simulink model "Quadcopter_nonlinear"  (R2023a)
settings: Solver=ode4  StartTime=0.0  StopTime=0.2  FixedStep=0.02  RelTol=1e-3
values from neighbouring files (symbols this model uses):
  b = 1.10794e-5    (= 1.10794e-05)    [QuadParameter.m]
  d = 3.2e-6    (= 3.2e-06)    [QuadParameter.m]
  d_cg = 0.295    [QuadParameter.m]
  Gamma1 = 4.98954110218396e-06    (= 4.98954110218e-06)    [final_PS.m]
  Gamma10 = -1.44562619785504e-05    (= -1.44562619786e-05)    [final_PS.m]
  Gamma11 = 24.4566929368231    (= 24.4566929368)    [final_PS.m]
  Gamma2 = 0.00290613207976024    (= 0.00290613207976)    [final_PS.m]
  Gamma3 = 42.1805100768496    (= 42.1805100768)    [final_PS.m]
  Gamma4 = 0.000237183411278011    (= 0.000237183411278)    [final_PS.m]
  Gamma5 = -0.00234577516229748    (= -0.0023457751623)    [final_PS.m]
  Gamma6 = 2.52935414320957    (= 2.52935414321)    [final_PS.m]
  Gamma7 = 0.000224057181768728    (= 0.000224057181769)    [final_PS.m]
  Gamma8 = 18.4688604256806    (= 18.4688604257)    [final_PS.m]
  Gamma9 = 0.00216966508125569    (= 0.00216966508126)    [final_PS.m]
  init_I = data_I(1, :)    [PS_I.m]
  init_II = data_II(1, :)    [PS_II.m]
  init_III = data_III(1, :)    [PS_III.m]
  init_IV = data_IV(1, :)    [PS_IV.m]
  init_IX = data_IX(1, :)    [PS_IX.m]
  init_V = data_V(1, :)    [PS_V.m]
  init_VI = data_VI(1, :)    [PS_VI.m]
  Omega_I = Omega(1, :)    [PS_I.m]
  Omega_II = Omega(1, :)    [PS_II.m]
  Omega_III = Omega(1, :)    [PS_III.m]
  Omega_IV = Omega(1, :)    [PS_IV.m]
  Omega_IX = Omega(1, :)    [PS_IX.m]
  Omega_V = Omega(1, :)    [PS_V.m]
  Omega_VI = Omega(1, :)    [PS_VI.m]
  Omega_VII = Omega(1, :)    [PS_VII.m]
  Omega_VIII = Omega(1, :)    [PS_VIII.m]
  Omega_X = Omega(1, :)    [PS_X.m]
undefined symbols (not defined in the file or in its folder): init_VII, init_VIII, init_X
(part 1 of 3)
settings Model: Creator=Ali  LastModifiedBy=Ali
settings SolverCC: AlgebraicLoopSolver=TrustRegion
settings OptimizationCC: ReuseModelBlockBuffer=off
settings DebuggingCC: UnconnectedInputMsg=warning  UnconnectedOutputMsg=warning  UnconnectedLineMsg=warning
settings ModelReferenceCC: EnableRefExpFcnMdlSchedulingChecks=on

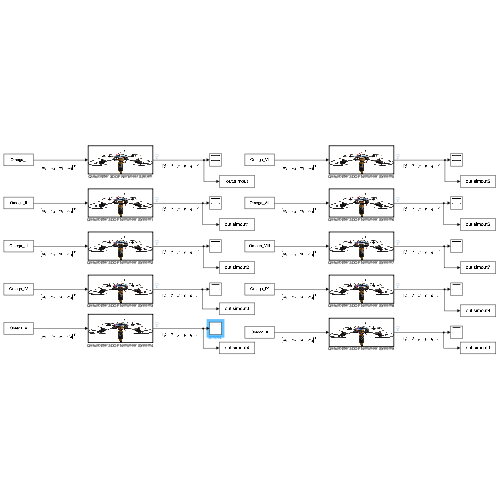
[thumbnail: Simulink's stored preview of the top-level diagram]
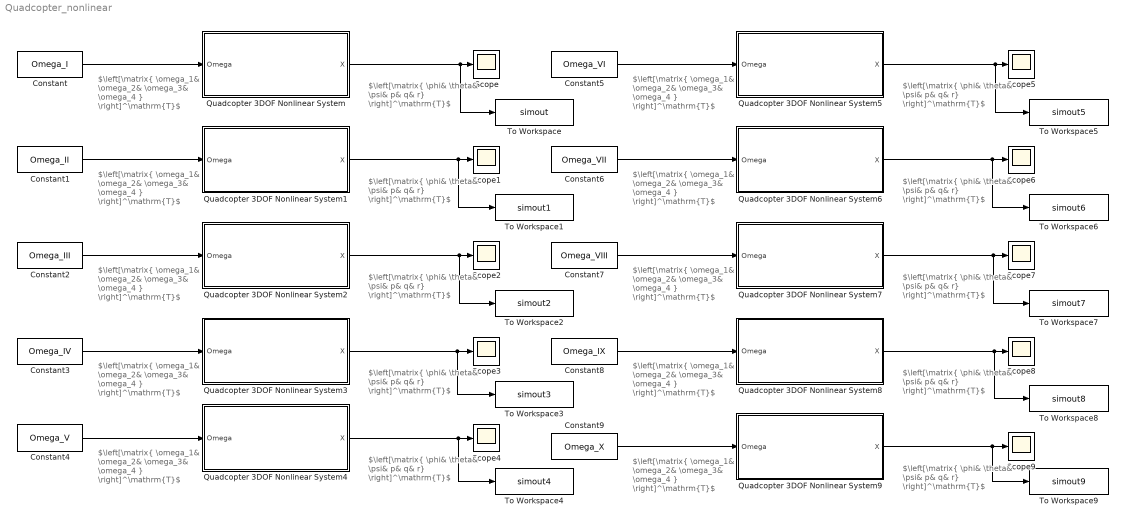
== system Quadcopter_nonlinear ==
  note: $\left[\matrix{ \omega_1& \omega_2& \omega_3& \omega_4 } \right]^\mathrm{T}$
  note: $\left[\matrix{ \phi& \theta& \psi& p& q& r} \right]^\mathrm{T}$
  note: $\left[\matrix{ \phi& \theta& \psi& p& q& r} \right]^\mathrm{T}$
  note: $\left[\matrix{ \omega_1& \omega_2& \omega_3& \omega_4 } \right]^\mathrm{T}$
  note: $\left[\matrix{ \phi& \theta& \psi& p& q& r} \right]^\mathrm{T}$
  note: $\left[\matrix{ \omega_1& \omega_2& \omega_3& \omega_4 } \right]^\mathrm{T}$
  note: $\left[\matrix{ \omega_1& \omega_2& \omega_3& \omega_4 } \right]^\mathrm{T}$
  note: $\left[\matrix{ \phi& \theta& \psi& p& q& r} \right]^\mathrm{T}$
  note: $\left[\matrix{ \phi& \theta& \psi& p& q& r} \right]^\mathrm{T}$
  note: $\left[\matrix{ \omega_1& \omega_2& \omega_3& \omega_4 } \right]^\mathrm{T}$
  note: $\left[\matrix{ \phi& \theta& \psi& p& q& r} \right]^\mathrm{T}$
  note: $\left[\matrix{ \phi& \theta& \psi& p& q& r} \right]^\mathrm{T}$
  note: $\left[\matrix{ \omega_1& \omega_2& \omega_3& \omega_4 } \right]^\mathrm{T}$
  note: $\left[\matrix{ \phi& \theta& \psi& p& q& r} \right]^\mathrm{T}$
  note: $\left[\matrix{ \phi& \theta& \psi& p& q& r} \right]^\mathrm{T}$
  note: $\left[\matrix{ \omega_1& \omega_2& \omega_3& \omega_4 } \right]^\mathrm{T}$
  note: $\left[\matrix{ \omega_1& \omega_2& \omega_3& \omega_4 } \right]^\mathrm{T}$
  note: $\left[\matrix{ \omega_1& \omega_2& \omega_3& \omega_4 } \right]^\mathrm{T}$
  note: $\left[\matrix{ \phi& \theta& \psi& p& q& r} \right]^\mathrm{T}$
  note: $\left[\matrix{ \omega_1& \omega_2& \omega_3& \omega_4 } \right]^\mathrm{T}$
  Constant : Constant  Value=Omega_I
  Constant1 : Constant  Value=Omega_II
  Constant2 : Constant  Value=Omega_III
  Constant3 : Constant  Value=Omega_IV
  Constant4 : Constant  Value=Omega_V
  Constant5 : Constant  Value=Omega_VI
  Constant6 : Constant  Value=Omega_VII
  Constant7 : Constant  Value=Omega_VIII
  Constant8 : Constant  Value=Omega_IX
  Constant9 : Constant  Value=Omega_X
  Quadcopter 3DOF Nonlinear System : Subsystem  TreatAsAtomicUnit=on
      mask Display: image('quad1.png'); % Use "Edit Image" on toolstrip to change.
  Quadcopter 3DOF Nonlinear System1 : Subsystem  TreatAsAtomicUnit=on
      mask Display: image('quad1.png'); % Use "Edit Image" on toolstrip to change.
  Quadcopter 3DOF Nonlinear System2 : Subsystem  TreatAsAtomicUnit=on
      mask Display: image('quad1.png'); % Use "Edit Image" on toolstrip to change.
  Quadcopter 3DOF Nonlinear System3 : Subsystem  TreatAsAtomicUnit=on
      mask Display: image('quad1.png'); % Use "Edit Image" on toolstrip to change.
  Quadcopter 3DOF Nonlinear System4 : Subsystem  TreatAsAtomicUnit=on
      mask Display: image('quad1.png'); % Use "Edit Image" on toolstrip to change.
  Quadcopter 3DOF Nonlinear System5 : Subsystem  TreatAsAtomicUnit=on
      mask Display: image('quad1.png'); % Use "Edit Image" on toolstrip to change.
  Quadcopter 3DOF Nonlinear System6 : Subsystem  TreatAsAtomicUnit=on
      mask Display: image('quad1.png'); % Use "Edit Image" on toolstrip to change.
  Quadcopter 3DOF Nonlinear System7 : Subsystem  TreatAsAtomicUnit=on
      mask Display: image('quad1.png'); % Use "Edit Image" on toolstrip to change.
  Quadcopter 3DOF Nonlinear System8 : Subsystem  TreatAsAtomicUnit=on
      mask Display: image('quad1.png'); % Use "Edit Image" on toolstrip to change.
  Quadcopter 3DOF Nonlinear System9 : Subsystem  TreatAsAtomicUnit=on
      mask Display: image('quad1.png'); % Use "Edit Image" on toolstrip to change.
  Scope{,1..9} (10 alike) : Scope
  To Workspace : ToWorkspace  VariableName=simout  SampleTime=-1
      settings: Save2DSignal=2-D array (concatenate along first dimension)
  To Workspace1 : ToWorkspace  VariableName=simout1  SampleTime=-1
      settings: Save2DSignal=2-D array (concatenate along first dimension)
  To Workspace2 : ToWorkspace  VariableName=simout2  SampleTime=-1
      settings: Save2DSignal=2-D array (concatenate along first dimension)
  To Workspace3 : ToWorkspace  VariableName=simout3  SampleTime=-1
      settings: Save2DSignal=2-D array (concatenate along first dimension)
  To Workspace4 : ToWorkspace  VariableName=simout4  SampleTime=-1
      settings: Save2DSignal=2-D array (concatenate along first dimension)
  To Workspace5 : ToWorkspace  VariableName=simout5  SampleTime=-1
      settings: Save2DSignal=2-D array (concatenate along first dimension)
  To Workspace6 : ToWorkspace  VariableName=simout6  SampleTime=-1
      settings: Save2DSignal=2-D array (concatenate along first dimension)
  To Workspace7 : ToWorkspace  VariableName=simout7  SampleTime=-1
      settings: Save2DSignal=2-D array (concatenate along first dimension)
  To Workspace8 : ToWorkspace  VariableName=simout8  SampleTime=-1
      settings: Save2DSignal=2-D array (concatenate along first dimension)
  To Workspace9 : ToWorkspace  VariableName=simout9  SampleTime=-1
      settings: Save2DSignal=2-D array (concatenate along first dimension)
  wires:
  Constant/1 -> Quadcopter 3DOF Nonlinear System/1(Omega)
  Quadcopter 3DOF Nonlinear System/1(X) -> To Workspace/1, Scope/1
  Constant1/1 -> Quadcopter 3DOF Nonlinear System1/1(Omega)
  Quadcopter 3DOF Nonlinear System1/1(X) -> To Workspace1/1, Scope1/1
  Constant2/1 -> Quadcopter 3DOF Nonlinear System2/1(Omega)
  Quadcopter 3DOF Nonlinear System2/1(X) -> To Workspace2/1, Scope2/1
  Quadcopter 3DOF Nonlinear System3/1(X) -> To Workspace3/1, Scope3/1
  Constant3/1 -> Quadcopter 3DOF Nonlinear System3/1(Omega)
  Quadcopter 3DOF Nonlinear System4/1(X) -> To Workspace4/1, Scope4/1
  Constant4/1 -> Quadcopter 3DOF Nonlinear System4/1(Omega)
  Constant5/1 -> Quadcopter 3DOF Nonlinear System5/1(Omega)
  Quadcopter 3DOF Nonlinear System8/1(X) -> To Workspace8/1, Scope8/1
  Quadcopter 3DOF Nonlinear System6/1(X) -> To Workspace6/1, Scope6/1
  Constant6/1 -> Quadcopter 3DOF Nonlinear System6/1(Omega)
  Quadcopter 3DOF Nonlinear System7/1(X) -> To Workspace7/1, Scope7/1
  Quadcopter 3DOF Nonlinear System5/1(X) -> To Workspace5/1, Scope5/1
  Constant7/1 -> Quadcopter 3DOF Nonlinear System7/1(Omega)
  Constant8/1 -> Quadcopter 3DOF Nonlinear System8/1(Omega)
  Quadcopter 3DOF Nonlinear System9/1(X) -> To Workspace9/1, Scope9/1
  Constant9/1 -> Quadcopter 3DOF Nonlinear System9/1(Omega)

== system Quadcopter_nonlinear/Quadcopter 3DOF Nonlinear System ==
  note: $\dot X$
  note: $\left[\matrix{ \dot\phi& \dot\theta& \dot\psi& \dot p& \dot q& \dot r} \right]^\mathrm{T}$
  note: $\left[\matrix{ \phi& \theta& \psi& p& q& r} \right]^\mathrm{T}$
  Omega : Inport
  Integrator : Integrator  InitialCondition=init_I
  Quad System1 : Subsystem
  X : Outport
  wires:
  Integrator/1 -> Quad System1/1(X), X/1  "X"
  Quad System1/1(dot(X)) -> Integrator/1  "dot(X)"
  Omega/1 -> Quad System1/2(Omega)

== system Quadcopter_nonlinear/Quadcopter 3DOF Nonlinear System1 ==
  note: $\dot X$
  note: $\left[\matrix{ \dot\phi& \dot\theta& \dot\psi& \dot p& \dot q& \dot r} \right]^\mathrm{T}$
  note: $\left[\matrix{ \phi& \theta& \psi& p& q& r} \right]^\mathrm{T}$
  Omega : Inport
  Integrator : Integrator  InitialCondition=init_II
  Quad System1 : Subsystem
  X : Outport
  wires:
  Integrator/1 -> Quad System1/1(X), X/1  "X"
  Quad System1/1(dot(X)) -> Integrator/1  "dot(X)"
  Omega/1 -> Quad System1/2(Omega)

== system Quadcopter_nonlinear/Quadcopter 3DOF Nonlinear System2 ==
  note: $\dot X$
  note: $\left[\matrix{ \dot\phi& \dot\theta& \dot\psi& \dot p& \dot q& \dot r} \right]^\mathrm{T}$
  note: $\left[\matrix{ \phi& \theta& \psi& p& q& r} \right]^\mathrm{T}$
  Omega : Inport
  Integrator : Integrator  InitialCondition=init_III
  Quad System1 : Subsystem
  X : Outport
  wires:
  Integrator/1 -> Quad System1/1(X), X/1  "X"
  Quad System1/1(dot(X)) -> Integrator/1  "dot(X)"
  Omega/1 -> Quad System1/2(Omega)

== system Quadcopter_nonlinear/Quadcopter 3DOF Nonlinear System3 ==
  note: $\dot X$
  note: $\left[\matrix{ \dot\phi& \dot\theta& \dot\psi& \dot p& \dot q& \dot r} \right]^\mathrm{T}$
  note: $\left[\matrix{ \phi& \theta& \psi& p& q& r} \right]^\mathrm{T}$
  Omega : Inport
  Integrator : Integrator  InitialCondition=init_IV
  Quad System1 : Subsystem
  X : Outport
  wires:
  Integrator/1 -> Quad System1/1(X), X/1  "X"
  Quad System1/1(dot(X)) -> Integrator/1  "dot(X)"
  Omega/1 -> Quad System1/2(Omega)

== system Quadcopter_nonlinear/Quadcopter 3DOF Nonlinear System4 ==
  note: $\dot X$
  note: $\left[\matrix{ \dot\phi& \dot\theta& \dot\psi& \dot p& \dot q& \dot r} \right]^\mathrm{T}$
  note: $\left[\matrix{ \phi& \theta& \psi& p& q& r} \right]^\mathrm{T}$
  Omega : Inport
  Integrator : Integrator  InitialCondition=init_V
  Quad System1 : Subsystem
  X : Outport
  wires:
  Integrator/1 -> Quad System1/1(X), X/1  "X"
  Quad System1/1(dot(X)) -> Integrator/1  "dot(X)"
  Omega/1 -> Quad System1/2(Omega)

== system Quadcopter_nonlinear/Quadcopter 3DOF Nonlinear System5 ==
  note: $\dot X$
  note: $\left[\matrix{ \dot\phi& \dot\theta& \dot\psi& \dot p& \dot q& \dot r} \right]^\mathrm{T}$
  note: $\left[\matrix{ \phi& \theta& \psi& p& q& r} \right]^\mathrm{T}$
  Omega : Inport
  Integrator : Integrator  InitialCondition=init_VI
  Quad System1 : Subsystem
  X : Outport
  wires:
  Integrator/1 -> Quad System1/1(X), X/1  "X"
  Quad System1/1(dot(X)) -> Integrator/1  "dot(X)"
  Omega/1 -> Quad System1/2(Omega)

== system Quadcopter_nonlinear/Quadcopter 3DOF Nonlinear System6 ==
  note: $\dot X$
  note: $\left[\matrix{ \dot\phi& \dot\theta& \dot\psi& \dot p& \dot q& \dot r} \right]^\mathrm{T}$
  note: $\left[\matrix{ \phi& \theta& \psi& p& q& r} \right]^\mathrm{T}$
  Omega : Inport
  Integrator : Integrator  InitialCondition=init_VII
  Quad System1 : Subsystem
  X : Outport
  wires:
  Integrator/1 -> Quad System1/1(X), X/1  "X"
  Quad System1/1(dot(X)) -> Integrator/1  "dot(X)"
  Omega/1 -> Quad System1/2(Omega)

== system Quadcopter_nonlinear/Quadcopter 3DOF Nonlinear System7 ==
  note: $\dot X$
  note: $\left[\matrix{ \dot\phi& \dot\theta& \dot\psi& \dot p& \dot q& \dot r} \right]^\mathrm{T}$
  note: $\left[\matrix{ \phi& \theta& \psi& p& q& r} \right]^\mathrm{T}$
  Omega : Inport
  Integrator : Integrator  InitialCondition=init_VIII
  Quad System1 : Subsystem
  X : Outport
  wires:
  Integrator/1 -> Quad System1/1(X), X/1  "X"
  Quad System1/1(dot(X)) -> Integrator/1  "dot(X)"
  Omega/1 -> Quad System1/2(Omega)

== system Quadcopter_nonlinear/Quadcopter 3DOF Nonlinear System8 ==
  note: $\dot X$
  note: $\left[\matrix{ \dot\phi& \dot\theta& \dot\psi& \dot p& \dot q& \dot r} \right]^\mathrm{T}$
  note: $\left[\matrix{ \phi& \theta& \psi& p& q& r} \right]^\mathrm{T}$
  Omega : Inport
  Integrator : Integrator  InitialCondition=init_IX
  Quad System1 : Subsystem
  X : Outport
  wires:
  Integrator/1 -> Quad System1/1(X), X/1  "X"
  Quad System1/1(dot(X)) -> Integrator/1  "dot(X)"
  Omega/1 -> Quad System1/2(Omega)

== system Quadcopter_nonlinear/Quadcopter 3DOF Nonlinear System9 ==
  note: $\dot X$
  note: $\left[\matrix{ \dot\phi& \dot\theta& \dot\psi& \dot p& \dot q& \dot r} \right]^\mathrm{T}$
  note: $\left[\matrix{ \phi& \theta& \psi& p& q& r} \right]^\mathrm{T}$
  Omega : Inport
  Integrator : Integrator  InitialCondition=init_X
  Quad System1 : Subsystem
  X : Outport
  wires:
  Integrator/1 -> Quad System1/1(X), X/1  "X"
  Quad System1/1(dot(X)) -> Integrator/1  "dot(X)"
  Omega/1 -> Quad System1/2(Omega)

== system Quadcopter_nonlinear/Quadcopter 3DOF Nonlinear System/Quad System1 ==
  X : Inport
  Omega : Inport  Port=2
  Quad System : Subsystem
  Selector : Selector  InputPortWidth=6  IndexOptions=Index vector (dialog)  Indices=[1 2 3 4 5 6]  OutputSizes=1
  Subsystem : Subsystem
  dot(X) : Outport
  wires:
  Selector/1 -> dot(X)/1  "dot(X)"
  X/1 -> Subsystem/1(X)
  Omega/1 -> Quad System/2(Omega)
  Quad System/1(dot(X)) -> Selector/1  "dot(X)"
  Subsystem/1(X_6) -> Quad System/1(X)

== system Quadcopter_nonlinear/Quadcopter 3DOF Nonlinear System1/Quad System1 ==
  X : Inport
  Omega : Inport  Port=2
  Quad System : Subsystem
  Selector : Selector  InputPortWidth=6  IndexOptions=Index vector (dialog)  Indices=[1 2 3 4 5 6]  OutputSizes=1
  Subsystem : Subsystem
  dot(X) : Outport
  wires:
  Selector/1 -> dot(X)/1  "dot(X)"
  X/1 -> Subsystem/1(X)
  Omega/1 -> Quad System/2(Omega)
  Quad System/1(dot(X)) -> Selector/1  "dot(X)"
  Subsystem/1(X_6) -> Quad System/1(X)

== system Quadcopter_nonlinear/Quadcopter 3DOF Nonlinear System2/Quad System1 ==
  X : Inport
  Omega : Inport  Port=2
  Quad System : Subsystem
  Selector : Selector  InputPortWidth=6  IndexOptions=Index vector (dialog)  Indices=[1 2 3 4 5 6]  OutputSizes=1
  Subsystem : Subsystem
  dot(X) : Outport
  wires:
  Selector/1 -> dot(X)/1  "dot(X)"
  X/1 -> Subsystem/1(X)
  Omega/1 -> Quad System/2(Omega)
  Quad System/1(dot(X)) -> Selector/1  "dot(X)"
  Subsystem/1(X_6) -> Quad System/1(X)

== system Quadcopter_nonlinear/Quadcopter 3DOF Nonlinear System3/Quad System1 ==
  X : Inport
  Omega : Inport  Port=2
  Quad System : Subsystem
  Selector : Selector  InputPortWidth=6  IndexOptions=Index vector (dialog)  Indices=[1 2 3 4 5 6]  OutputSizes=1
  Subsystem : Subsystem
  dot(X) : Outport
  wires:
  Selector/1 -> dot(X)/1  "dot(X)"
  X/1 -> Subsystem/1(X)
  Omega/1 -> Quad System/2(Omega)
  Quad System/1(dot(X)) -> Selector/1  "dot(X)"
  Subsystem/1(X_6) -> Quad System/1(X)

== system Quadcopter_nonlinear/Quadcopter 3DOF Nonlinear System4/Quad System1 ==
  X : Inport
  Omega : Inport  Port=2
  Quad System : Subsystem
  Selector : Selector  InputPortWidth=6  IndexOptions=Index vector (dialog)  Indices=[1 2 3 4 5 6]  OutputSizes=1
  Subsystem : Subsystem
  dot(X) : Outport
  wires:
  Selector/1 -> dot(X)/1  "dot(X)"
  X/1 -> Subsystem/1(X)
  Omega/1 -> Quad System/2(Omega)
  Quad System/1(dot(X)) -> Selector/1  "dot(X)"
  Subsystem/1(X_6) -> Quad System/1(X)

== system Quadcopter_nonlinear/Quadcopter 3DOF Nonlinear System5/Quad System1 ==
  X : Inport
  Omega : Inport  Port=2
  Quad System : Subsystem
  Selector : Selector  InputPortWidth=6  IndexOptions=Index vector (dialog)  Indices=[1 2 3 4 5 6]  OutputSizes=1
  Subsystem : Subsystem
  dot(X) : Outport
  wires:
  Selector/1 -> dot(X)/1  "dot(X)"
  X/1 -> Subsystem/1(X)
  Omega/1 -> Quad System/2(Omega)
  Quad System/1(dot(X)) -> Selector/1  "dot(X)"
  Subsystem/1(X_6) -> Quad System/1(X)

== system Quadcopter_nonlinear/Quadcopter 3DOF Nonlinear System6/Quad System1 ==
  X : Inport
  Omega : Inport  Port=2
  Quad System : Subsystem
  Selector : Selector  InputPortWidth=6  IndexOptions=Index vector (dialog)  Indices=[1 2 3 4 5 6]  OutputSizes=1
  Subsystem : Subsystem
  dot(X) : Outport
  wires:
  Selector/1 -> dot(X)/1  "dot(X)"
  X/1 -> Subsystem/1(X)
  Omega/1 -> Quad System/2(Omega)
  Quad System/1(dot(X)) -> Selector/1  "dot(X)"
  Subsystem/1(X_6) -> Quad System/1(X)

== system Quadcopter_nonlinear/Quadcopter 3DOF Nonlinear System7/Quad System1 ==
  X : Inport
  Omega : Inport  Port=2
  Quad System : Subsystem
  Selector : Selector  InputPortWidth=6  IndexOptions=Index vector (dialog)  Indices=[1 2 3 4 5 6]  OutputSizes=1
  Subsystem : Subsystem
  dot(X) : Outport
  wires:
  Selector/1 -> dot(X)/1  "dot(X)"
  X/1 -> Subsystem/1(X)
  Omega/1 -> Quad System/2(Omega)
  Quad System/1(dot(X)) -> Selector/1  "dot(X)"
  Subsystem/1(X_6) -> Quad System/1(X)

== system Quadcopter_nonlinear/Quadcopter 3DOF Nonlinear System8/Quad System1 ==
  X : Inport
  Omega : Inport  Port=2
  Quad System : Subsystem
  Selector : Selector  InputPortWidth=6  IndexOptions=Index vector (dialog)  Indices=[1 2 3 4 5 6]  OutputSizes=1
  Subsystem : Subsystem
  dot(X) : Outport
  wires:
  Selector/1 -> dot(X)/1  "dot(X)"
  X/1 -> Subsystem/1(X)
  Omega/1 -> Quad System/2(Omega)
  Quad System/1(dot(X)) -> Selector/1  "dot(X)"
  Subsystem/1(X_6) -> Quad System/1(X)

== system Quadcopter_nonlinear/Quadcopter 3DOF Nonlinear System9/Quad System1 ==
  X : Inport
  Omega : Inport  Port=2
  Quad System : Subsystem
  Selector : Selector  InputPortWidth=6  IndexOptions=Index vector (dialog)  Indices=[1 2 3 4 5 6]  OutputSizes=1
  Subsystem : Subsystem
  dot(X) : Outport
  wires:
  Selector/1 -> dot(X)/1  "dot(X)"
  X/1 -> Subsystem/1(X)
  Omega/1 -> Quad System/2(Omega)
  Quad System/1(dot(X)) -> Selector/1  "dot(X)"
  Subsystem/1(X_6) -> Quad System/1(X)

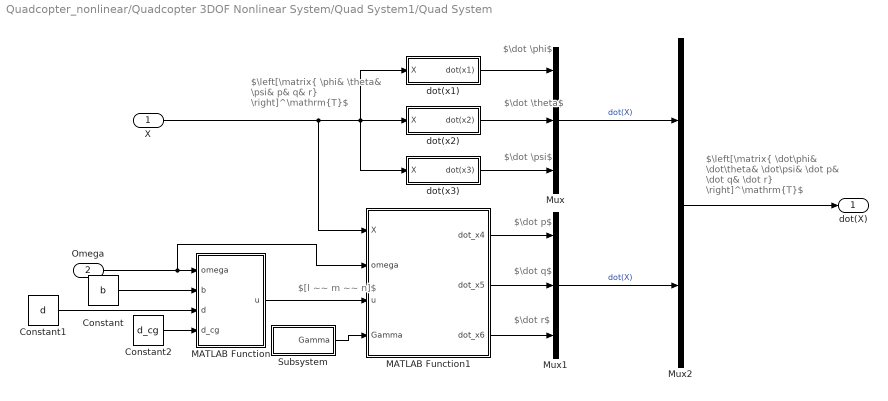
== system Quadcopter_nonlinear/Quadcopter 3DOF Nonlinear System/Quad System1/Quad System ==
  note: $\dot \phi$
  note: $\left[\matrix{ \phi& \theta& \psi& p& q& r} \right]^\mathrm{T}$
  note: $[l ~~ m ~~ n]$
  note: $\dot \theta$
  note: $\dot \psi$
  note: $\dot p$
  note: $\dot q$
  note: $\dot r$
  note: $\left[\matrix{ \dot\phi& \dot\theta& \dot\psi& \dot p& \dot q& \dot r} \right]^\mathrm{T}$
  X : Inport
  Omega : Inport  Port=2
  Constant : Constant  Value=b
  Constant1 : Constant  Value=d
  Constant2 : Constant  Value=d_cg
  MATLAB Function : MATLAB Function  TreatAsAtomicUnit=on
  MATLAB Function1 : MATLAB Function  TreatAsAtomicUnit=on
  Mux : Mux  Inputs=3
  Mux1 : Mux  Inputs=3
  Mux2 : Mux  Inputs=2
  Subsystem : Subsystem
  dot(x1) : Subsystem
  dot(x2) : Subsystem
  dot(x3) : Subsystem
  dot(X) : Outport
  wires:
  X/1 -> MATLAB Function1/1(X), dot(x3)/1(X), dot(x1)/1(X), dot(x2)/1(X)
  Omega/1 -> MATLAB Function1/2(omega), MATLAB Function/1(omega)
  MATLAB Function1/2(dot_x5) -> Mux1/2
  dot(x2)/1(dot(x2)) -> Mux/2
  MATLAB Function1/1(dot_x4) -> Mux1/1
  dot(x3)/1(dot(x3)) -> Mux/3
  dot(x1)/1(dot(x1)) -> Mux/1
  MATLAB Function1/3(dot_x6) -> Mux1/3
  Constant/1 -> MATLAB Function/2(b)
  Constant1/1 -> MATLAB Function/3(d)
  MATLAB Function/1(u) -> MATLAB Function1/3(u)
  Mux1/1 -> Mux2/2  "dot(X)"
  Mux/1 -> Mux2/1  "dot(X)"
  Mux2/1 -> dot(X)/1
  Subsystem/1(Gamma) -> MATLAB Function1/4(Gamma)
  Constant2/1 -> MATLAB Function/4(d_cg)

== system Quadcopter_nonlinear/Quadcopter 3DOF Nonlinear System/Quad System1/Subsystem ==
  X : Inport
  Mux : Mux  Inputs=6
  Selector1 : Selector  InputPortWidth=6  IndexOptions=Index vector (dialog)  Indices=[1]  OutputSizes=1
  Selector2 : Selector  InputPortWidth=6  IndexOptions=Index vector (dialog)  Indices=[4]  OutputSizes=1
  Selector3 : Selector  InputPortWidth=6  IndexOptions=Index vector (dialog)  Indices=[2]  OutputSizes=1
  Selector4 : Selector  InputPortWidth=6  IndexOptions=Index vector (dialog)  Indices=[5]  OutputSizes=1
  Selector5 : Selector  InputPortWidth=6  IndexOptions=Index vector (dialog)  Indices=[3]  OutputSizes=1
  Selector6 : Selector  InputPortWidth=6  IndexOptions=Index vector (dialog)  Indices=[6]  OutputSizes=1
  X_6 : Outport
  wires:
  Selector6/1 -> Mux/6
  Selector5/1 -> Mux/3
  Mux/1 -> X_6/1
  Selector3/1 -> Mux/2
  Selector2/1 -> Mux/4
  Selector1/1 -> Mux/1
  Selector4/1 -> Mux/5
  X/1 -> Selector3/1, Selector5/1, Selector6/1, Selector4/1, Selector2/1, Selector1/1

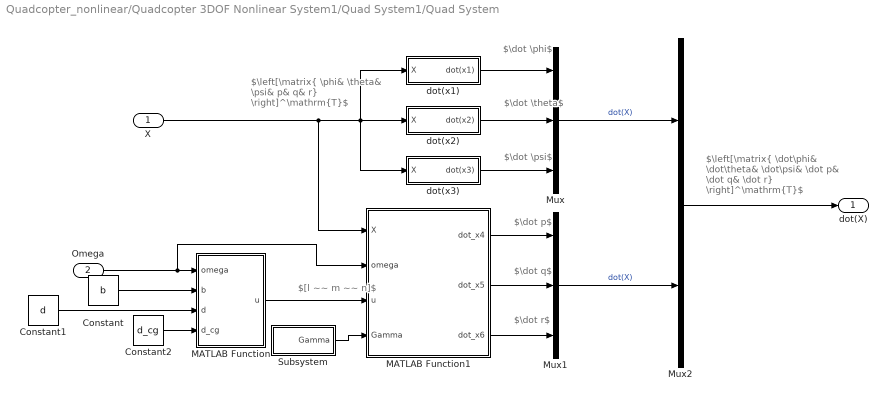
== system Quadcopter_nonlinear/Quadcopter 3DOF Nonlinear System1/Quad System1/Quad System ==
  note: $\dot \phi$
  note: $\left[\matrix{ \phi& \theta& \psi& p& q& r} \right]^\mathrm{T}$
  note: $[l ~~ m ~~ n]$
  note: $\dot \theta$
  note: $\dot \psi$
  note: $\dot p$
  note: $\dot q$
  note: $\dot r$
  note: $\left[\matrix{ \dot\phi& \dot\theta& \dot\psi& \dot p& \dot q& \dot r} \right]^\mathrm{T}$
  X : Inport
  Omega : Inport  Port=2
  Constant : Constant  Value=b
  Constant1 : Constant  Value=d
  Constant2 : Constant  Value=d_cg
  MATLAB Function : MATLAB Function  TreatAsAtomicUnit=on
  MATLAB Function1 : MATLAB Function  TreatAsAtomicUnit=on
  Mux : Mux  Inputs=3
  Mux1 : Mux  Inputs=3
  Mux2 : Mux  Inputs=2
  Subsystem : Subsystem
  dot(x1) : Subsystem
  dot(x2) : Subsystem
  dot(x3) : Subsystem
  dot(X) : Outport
  wires:
  X/1 -> MATLAB Function1/1(X), dot(x3)/1(X), dot(x1)/1(X), dot(x2)/1(X)
  Omega/1 -> MATLAB Function1/2(omega), MATLAB Function/1(omega)
  MATLAB Function1/2(dot_x5) -> Mux1/2
  dot(x2)/1(dot(x2)) -> Mux/2
  MATLAB Function1/1(dot_x4) -> Mux1/1
  dot(x3)/1(dot(x3)) -> Mux/3
  dot(x1)/1(dot(x1)) -> Mux/1
  MATLAB Function1/3(dot_x6) -> Mux1/3
  Constant/1 -> MATLAB Function/2(b)
  Constant1/1 -> MATLAB Function/3(d)
  MATLAB Function/1(u) -> MATLAB Function1/3(u)
  Mux1/1 -> Mux2/2  "dot(X)"
  Mux/1 -> Mux2/1  "dot(X)"
  Mux2/1 -> dot(X)/1
  Subsystem/1(Gamma) -> MATLAB Function1/4(Gamma)
  Constant2/1 -> MATLAB Function/4(d_cg)

== system Quadcopter_nonlinear/Quadcopter 3DOF Nonlinear System1/Quad System1/Subsystem ==
  X : Inport
  Mux : Mux  Inputs=6
  Selector1 : Selector  InputPortWidth=6  IndexOptions=Index vector (dialog)  Indices=[1]  OutputSizes=1
  Selector2 : Selector  InputPortWidth=6  IndexOptions=Index vector (dialog)  Indices=[4]  OutputSizes=1
  Selector3 : Selector  InputPortWidth=6  IndexOptions=Index vector (dialog)  Indices=[2]  OutputSizes=1
  Selector4 : Selector  InputPortWidth=6  IndexOptions=Index vector (dialog)  Indices=[5]  OutputSizes=1
  Selector5 : Selector  InputPortWidth=6  IndexOptions=Index vector (dialog)  Indices=[3]  OutputSizes=1
  Selector6 : Selector  InputPortWidth=6  IndexOptions=Index vector (dialog)  Indices=[6]  OutputSizes=1
  X_6 : Outport
  wires:
  Selector6/1 -> Mux/6
  Selector5/1 -> Mux/3
  Mux/1 -> X_6/1
  Selector3/1 -> Mux/2
  Selector2/1 -> Mux/4
  Selector1/1 -> Mux/1
  Selector4/1 -> Mux/5
  X/1 -> Selector3/1, Selector5/1, Selector6/1, Selector4/1, Selector2/1, Selector1/1

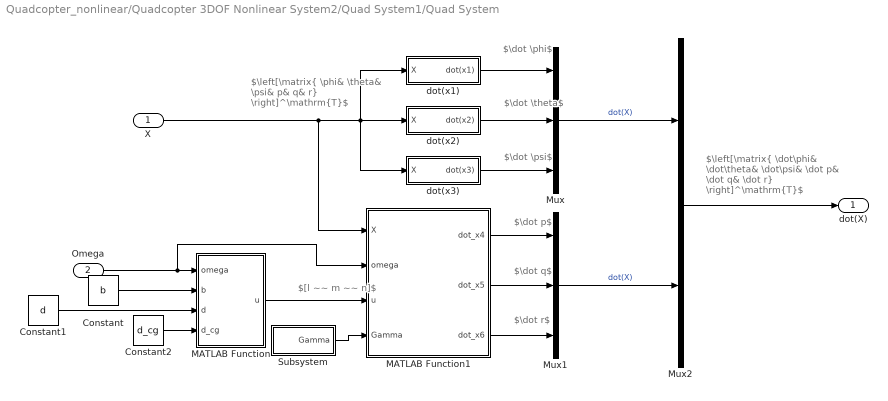
== system Quadcopter_nonlinear/Quadcopter 3DOF Nonlinear System2/Quad System1/Quad System ==
  note: $\dot \phi$
  note: $\left[\matrix{ \phi& \theta& \psi& p& q& r} \right]^\mathrm{T}$
  note: $[l ~~ m ~~ n]$
  note: $\dot \theta$
  note: $\dot \psi$
  note: $\dot p$
  note: $\dot q$
  note: $\dot r$
  note: $\left[\matrix{ \dot\phi& \dot\theta& \dot\psi& \dot p& \dot q& \dot r} \right]^\mathrm{T}$
  X : Inport
  Omega : Inport  Port=2
  Constant : Constant  Value=b
  Constant1 : Constant  Value=d
  Constant2 : Constant  Value=d_cg
  MATLAB Function : MATLAB Function  TreatAsAtomicUnit=on
  MATLAB Function1 : MATLAB Function  TreatAsAtomicUnit=on
  Mux : Mux  Inputs=3
  Mux1 : Mux  Inputs=3
  Mux2 : Mux  Inputs=2
  Subsystem : Subsystem
  dot(x1) : Subsystem
  dot(x2) : Subsystem
  dot(x3) : Subsystem
  dot(X) : Outport
  wires:
  X/1 -> MATLAB Function1/1(X), dot(x3)/1(X), dot(x1)/1(X), dot(x2)/1(X)
  Omega/1 -> MATLAB Function1/2(omega), MATLAB Function/1(omega)
  MATLAB Function1/2(dot_x5) -> Mux1/2
  dot(x2)/1(dot(x2)) -> Mux/2
  MATLAB Function1/1(dot_x4) -> Mux1/1
  dot(x3)/1(dot(x3)) -> Mux/3
  dot(x1)/1(dot(x1)) -> Mux/1
  MATLAB Function1/3(dot_x6) -> Mux1/3
  Constant/1 -> MATLAB Function/2(b)
  Constant1/1 -> MATLAB Function/3(d)
  MATLAB Function/1(u) -> MATLAB Function1/3(u)
  Mux1/1 -> Mux2/2  "dot(X)"
  Mux/1 -> Mux2/1  "dot(X)"
  Mux2/1 -> dot(X)/1
  Subsystem/1(Gamma) -> MATLAB Function1/4(Gamma)
  Constant2/1 -> MATLAB Function/4(d_cg)

== system Quadcopter_nonlinear/Quadcopter 3DOF Nonlinear System2/Quad System1/Subsystem ==
  X : Inport
  Mux : Mux  Inputs=6
  Selector1 : Selector  InputPortWidth=6  IndexOptions=Index vector (dialog)  Indices=[1]  OutputSizes=1
  Selector2 : Selector  InputPortWidth=6  IndexOptions=Index vector (dialog)  Indices=[4]  OutputSizes=1
  Selector3 : Selector  InputPortWidth=6  IndexOptions=Index vector (dialog)  Indices=[2]  OutputSizes=1
  Selector4 : Selector  InputPortWidth=6  IndexOptions=Index vector (dialog)  Indices=[5]  OutputSizes=1
  Selector5 : Selector  InputPortWidth=6  IndexOptions=Index vector (dialog)  Indices=[3]  OutputSizes=1
  Selector6 : Selector  InputPortWidth=6  IndexOptions=Index vector (dialog)  Indices=[6]  OutputSizes=1
  X_6 : Outport
  wires:
  Selector6/1 -> Mux/6
  Selector5/1 -> Mux/3
  Mux/1 -> X_6/1
  Selector3/1 -> Mux/2
  Selector2/1 -> Mux/4
  Selector1/1 -> Mux/1
  Selector4/1 -> Mux/5
  X/1 -> Selector3/1, Selector5/1, Selector6/1, Selector4/1, Selector2/1, Selector1/1

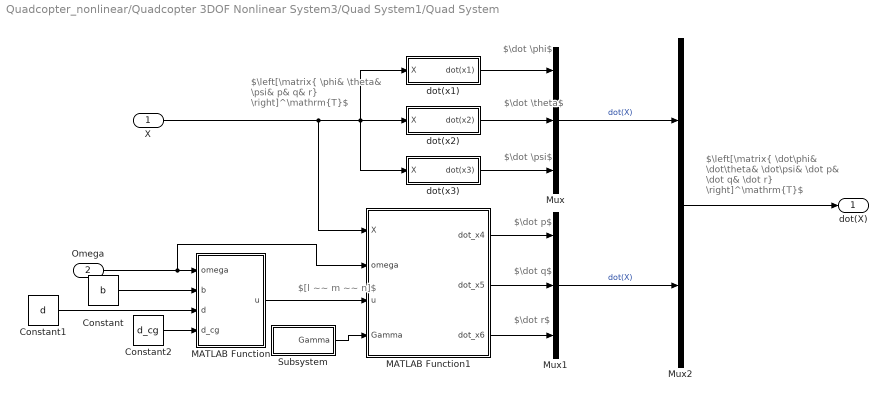
== system Quadcopter_nonlinear/Quadcopter 3DOF Nonlinear System3/Quad System1/Quad System ==
  note: $\dot \phi$
  note: $\left[\matrix{ \phi& \theta& \psi& p& q& r} \right]^\mathrm{T}$
  note: $[l ~~ m ~~ n]$
  note: $\dot \theta$
  note: $\dot \psi$
  note: $\dot p$
  note: $\dot q$
  note: $\dot r$
  note: $\left[\matrix{ \dot\phi& \dot\theta& \dot\psi& \dot p& \dot q& \dot r} \right]^\mathrm{T}$
  X : Inport
  Omega : Inport  Port=2
  Constant : Constant  Value=b
  Constant1 : Constant  Value=d
  Constant2 : Constant  Value=d_cg
  MATLAB Function : MATLAB Function  TreatAsAtomicUnit=on
  MATLAB Function1 : MATLAB Function  TreatAsAtomicUnit=on
  Mux : Mux  Inputs=3
  Mux1 : Mux  Inputs=3
  Mux2 : Mux  Inputs=2
  Subsystem : Subsystem
  dot(x1) : Subsystem
  dot(x2) : Subsystem
  dot(x3) : Subsystem
  dot(X) : Outport
  wires:
  X/1 -> MATLAB Function1/1(X), dot(x3)/1(X), dot(x1)/1(X), dot(x2)/1(X)
  Omega/1 -> MATLAB Function1/2(omega), MATLAB Function/1(omega)
  MATLAB Function1/2(dot_x5) -> Mux1/2
  dot(x2)/1(dot(x2)) -> Mux/2
  MATLAB Function1/1(dot_x4) -> Mux1/1
  dot(x3)/1(dot(x3)) -> Mux/3
  dot(x1)/1(dot(x1)) -> Mux/1
  MATLAB Function1/3(dot_x6) -> Mux1/3
  Constant/1 -> MATLAB Function/2(b)
  Constant1/1 -> MATLAB Function/3(d)
  MATLAB Function/1(u) -> MATLAB Function1/3(u)
  Mux1/1 -> Mux2/2  "dot(X)"
  Mux/1 -> Mux2/1  "dot(X)"
  Mux2/1 -> dot(X)/1
  Subsystem/1(Gamma) -> MATLAB Function1/4(Gamma)
  Constant2/1 -> MATLAB Function/4(d_cg)

== system Quadcopter_nonlinear/Quadcopter 3DOF Nonlinear System3/Quad System1/Subsystem ==
  X : Inport
  Mux : Mux  Inputs=6
  Selector1 : Selector  InputPortWidth=6  IndexOptions=Index vector (dialog)  Indices=[1]  OutputSizes=1
  Selector2 : Selector  InputPortWidth=6  IndexOptions=Index vector (dialog)  Indices=[4]  OutputSizes=1
  Selector3 : Selector  InputPortWidth=6  IndexOptions=Index vector (dialog)  Indices=[2]  OutputSizes=1
  Selector4 : Selector  InputPortWidth=6  IndexOptions=Index vector (dialog)  Indices=[5]  OutputSizes=1
  Selector5 : Selector  InputPortWidth=6  IndexOptions=Index vector (dialog)  Indices=[3]  OutputSizes=1
  Selector6 : Selector  InputPortWidth=6  IndexOptions=Index vector (dialog)  Indices=[6]  OutputSizes=1
  X_6 : Outport
  wires:
  Selector6/1 -> Mux/6
  Selector5/1 -> Mux/3
  Mux/1 -> X_6/1
  Selector3/1 -> Mux/2
  Selector2/1 -> Mux/4
  Selector1/1 -> Mux/1
  Selector4/1 -> Mux/5
  X/1 -> Selector3/1, Selector5/1, Selector6/1, Selector4/1, Selector2/1, Selector1/1

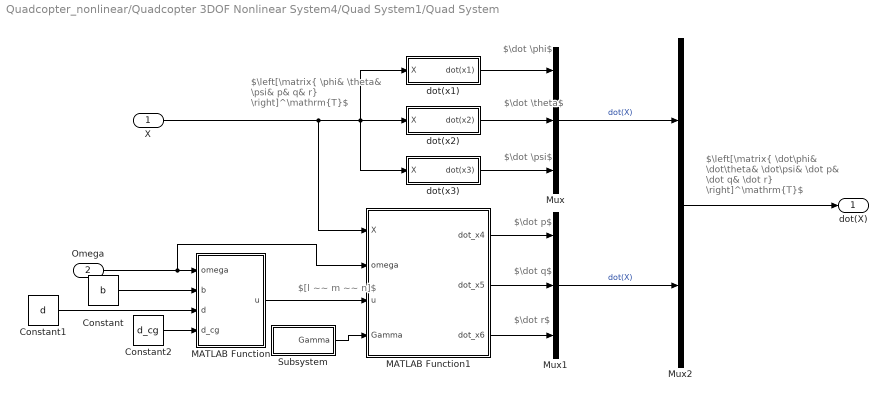
== system Quadcopter_nonlinear/Quadcopter 3DOF Nonlinear System4/Quad System1/Quad System ==
  note: $\dot \phi$
  note: $\left[\matrix{ \phi& \theta& \psi& p& q& r} \right]^\mathrm{T}$
  note: $[l ~~ m ~~ n]$
  note: $\dot \theta$
  note: $\dot \psi$
  note: $\dot p$
  note: $\dot q$
  note: $\dot r$
  note: $\left[\matrix{ \dot\phi& \dot\theta& \dot\psi& \dot p& \dot q& \dot r} \right]^\mathrm{T}$
  X : Inport
  Omega : Inport  Port=2
  Constant : Constant  Value=b
  Constant1 : Constant  Value=d
  Constant2 : Constant  Value=d_cg
  MATLAB Function : MATLAB Function  TreatAsAtomicUnit=on
  MATLAB Function1 : MATLAB Function  TreatAsAtomicUnit=on
  Mux : Mux  Inputs=3
  Mux1 : Mux  Inputs=3
  Mux2 : Mux  Inputs=2
  Subsystem : Subsystem
  dot(x1) : Subsystem
  dot(x2) : Subsystem
  dot(x3) : Subsystem
  dot(X) : Outport
  wires:
  X/1 -> MATLAB Function1/1(X), dot(x3)/1(X), dot(x1)/1(X), dot(x2)/1(X)
  Omega/1 -> MATLAB Function1/2(omega), MATLAB Function/1(omega)
  MATLAB Function1/2(dot_x5) -> Mux1/2
  dot(x2)/1(dot(x2)) -> Mux/2
  MATLAB Function1/1(dot_x4) -> Mux1/1
  dot(x3)/1(dot(x3)) -> Mux/3
  dot(x1)/1(dot(x1)) -> Mux/1
  MATLAB Function1/3(dot_x6) -> Mux1/3
  Constant/1 -> MATLAB Function/2(b)
  Constant1/1 -> MATLAB Function/3(d)
  MATLAB Function/1(u) -> MATLAB Function1/3(u)
  Mux1/1 -> Mux2/2  "dot(X)"
  Mux/1 -> Mux2/1  "dot(X)"
  Mux2/1 -> dot(X)/1
  Subsystem/1(Gamma) -> MATLAB Function1/4(Gamma)
  Constant2/1 -> MATLAB Function/4(d_cg)

== system Quadcopter_nonlinear/Quadcopter 3DOF Nonlinear System4/Quad System1/Subsystem ==
  X : Inport
  Mux : Mux  Inputs=6
  Selector1 : Selector  InputPortWidth=6  IndexOptions=Index vector (dialog)  Indices=[1]  OutputSizes=1
  Selector2 : Selector  InputPortWidth=6  IndexOptions=Index vector (dialog)  Indices=[4]  OutputSizes=1
  Selector3 : Selector  InputPortWidth=6  IndexOptions=Index vector (dialog)  Indices=[2]  OutputSizes=1
  Selector4 : Selector  InputPortWidth=6  IndexOptions=Index vector (dialog)  Indices=[5]  OutputSizes=1
  Selector5 : Selector  InputPortWidth=6  IndexOptions=Index vector (dialog)  Indices=[3]  OutputSizes=1
  Selector6 : Selector  InputPortWidth=6  IndexOptions=Index vector (dialog)  Indices=[6]  OutputSizes=1
  X_6 : Outport
  wires:
  Selector6/1 -> Mux/6
  Selector5/1 -> Mux/3
  Mux/1 -> X_6/1
  Selector3/1 -> Mux/2
  Selector2/1 -> Mux/4
  Selector1/1 -> Mux/1
  Selector4/1 -> Mux/5
  X/1 -> Selector3/1, Selector5/1, Selector6/1, Selector4/1, Selector2/1, Selector1/1

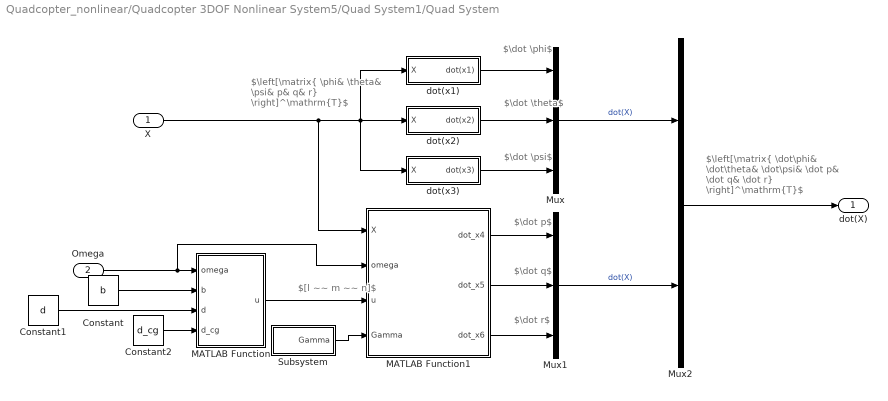
== system Quadcopter_nonlinear/Quadcopter 3DOF Nonlinear System5/Quad System1/Quad System ==
  note: $\dot \phi$
  note: $\left[\matrix{ \phi& \theta& \psi& p& q& r} \right]^\mathrm{T}$
  note: $[l ~~ m ~~ n]$
  note: $\dot \theta$
  note: $\dot \psi$
  note: $\dot p$
  note: $\dot q$
  note: $\dot r$
  note: $\left[\matrix{ \dot\phi& \dot\theta& \dot\psi& \dot p& \dot q& \dot r} \right]^\mathrm{T}$
  X : Inport
  Omega : Inport  Port=2
  Constant : Constant  Value=b
  Constant1 : Constant  Value=d
  Constant2 : Constant  Value=d_cg
  MATLAB Function : MATLAB Function  TreatAsAtomicUnit=on
  MATLAB Function1 : MATLAB Function  TreatAsAtomicUnit=on
  Mux : Mux  Inputs=3
  Mux1 : Mux  Inputs=3
  Mux2 : Mux  Inputs=2
  Subsystem : Subsystem
  dot(x1) : Subsystem
  dot(x2) : Subsystem
  dot(x3) : Subsystem
  dot(X) : Outport
  wires:
  X/1 -> MATLAB Function1/1(X), dot(x3)/1(X), dot(x1)/1(X), dot(x2)/1(X)
  Omega/1 -> MATLAB Function1/2(omega), MATLAB Function/1(omega)
  MATLAB Function1/2(dot_x5) -> Mux1/2
  dot(x2)/1(dot(x2)) -> Mux/2
  MATLAB Function1/1(dot_x4) -> Mux1/1
  dot(x3)/1(dot(x3)) -> Mux/3
  dot(x1)/1(dot(x1)) -> Mux/1
  MATLAB Function1/3(dot_x6) -> Mux1/3
  Constant/1 -> MATLAB Function/2(b)
  Constant1/1 -> MATLAB Function/3(d)
  MATLAB Function/1(u) -> MATLAB Function1/3(u)
  Mux1/1 -> Mux2/2  "dot(X)"
  Mux/1 -> Mux2/1  "dot(X)"
  Mux2/1 -> dot(X)/1
  Subsystem/1(Gamma) -> MATLAB Function1/4(Gamma)
  Constant2/1 -> MATLAB Function/4(d_cg)

== system Quadcopter_nonlinear/Quadcopter 3DOF Nonlinear System5/Quad System1/Subsystem ==
  X : Inport
  Mux : Mux  Inputs=6
  Selector1 : Selector  InputPortWidth=6  IndexOptions=Index vector (dialog)  Indices=[1]  OutputSizes=1
  Selector2 : Selector  InputPortWidth=6  IndexOptions=Index vector (dialog)  Indices=[4]  OutputSizes=1
  Selector3 : Selector  InputPortWidth=6  IndexOptions=Index vector (dialog)  Indices=[2]  OutputSizes=1
  Selector4 : Selector  InputPortWidth=6  IndexOptions=Index vector (dialog)  Indices=[5]  OutputSizes=1
  Selector5 : Selector  InputPortWidth=6  IndexOptions=Index vector (dialog)  Indices=[3]  OutputSizes=1
  Selector6 : Selector  InputPortWidth=6  IndexOptions=Index vector (dialog)  Indices=[6]  OutputSizes=1
  X_6 : Outport
  wires:
  Selector6/1 -> Mux/6
  Selector5/1 -> Mux/3
  Mux/1 -> X_6/1
  Selector3/1 -> Mux/2
  Selector2/1 -> Mux/4
  Selector1/1 -> Mux/1
  Selector4/1 -> Mux/5
  X/1 -> Selector3/1, Selector5/1, Selector6/1, Selector4/1, Selector2/1, Selector1/1

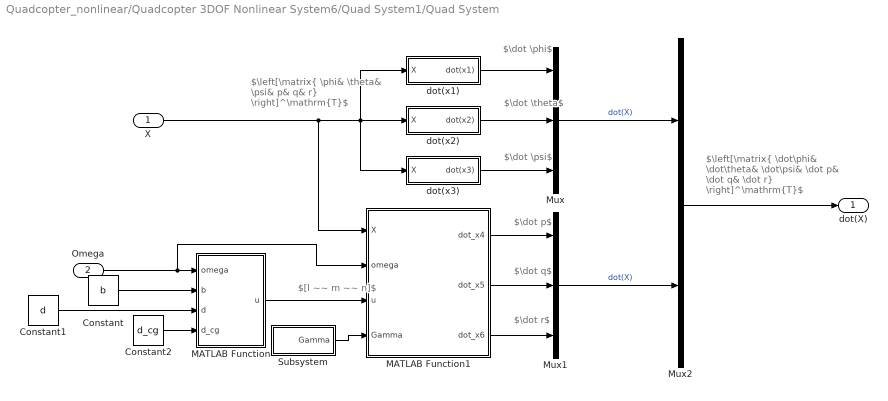
== system Quadcopter_nonlinear/Quadcopter 3DOF Nonlinear System6/Quad System1/Quad System ==
  note: $\dot \phi$
  note: $\left[\matrix{ \phi& \theta& \psi& p& q& r} \right]^\mathrm{T}$
  note: $[l ~~ m ~~ n]$
  note: $\dot \theta$
  note: $\dot \psi$
  note: $\dot p$
  note: $\dot q$
  note: $\dot r$
  note: $\left[\matrix{ \dot\phi& \dot\theta& \dot\psi& \dot p& \dot q& \dot r} \right]^\mathrm{T}$
  X : Inport
  Omega : Inport  Port=2
  Constant : Constant  Value=b
  Constant1 : Constant  Value=d
  Constant2 : Constant  Value=d_cg
  MATLAB Function : MATLAB Function  TreatAsAtomicUnit=on
  MATLAB Function1 : MATLAB Function  TreatAsAtomicUnit=on
  Mux : Mux  Inputs=3
  Mux1 : Mux  Inputs=3
  Mux2 : Mux  Inputs=2
  Subsystem : Subsystem
  dot(x1) : Subsystem
  dot(x2) : Subsystem
  dot(x3) : Subsystem
  dot(X) : Outport
  wires:
  X/1 -> MATLAB Function1/1(X), dot(x3)/1(X), dot(x1)/1(X), dot(x2)/1(X)
  Omega/1 -> MATLAB Function1/2(omega), MATLAB Function/1(omega)
  MATLAB Function1/2(dot_x5) -> Mux1/2
  dot(x2)/1(dot(x2)) -> Mux/2
  MATLAB Function1/1(dot_x4) -> Mux1/1
  dot(x3)/1(dot(x3)) -> Mux/3
  dot(x1)/1(dot(x1)) -> Mux/1
  MATLAB Function1/3(dot_x6) -> Mux1/3
  Constant/1 -> MATLAB Function/2(b)
  Constant1/1 -> MATLAB Function/3(d)
  MATLAB Function/1(u) -> MATLAB Function1/3(u)
  Mux1/1 -> Mux2/2  "dot(X)"
  Mux/1 -> Mux2/1  "dot(X)"
  Mux2/1 -> dot(X)/1
  Subsystem/1(Gamma) -> MATLAB Function1/4(Gamma)
  Constant2/1 -> MATLAB Function/4(d_cg)

== system Quadcopter_nonlinear/Quadcopter 3DOF Nonlinear System6/Quad System1/Subsystem ==
  X : Inport
  Mux : Mux  Inputs=6
  Selector1 : Selector  InputPortWidth=6  IndexOptions=Index vector (dialog)  Indices=[1]  OutputSizes=1
  Selector2 : Selector  InputPortWidth=6  IndexOptions=Index vector (dialog)  Indices=[4]  OutputSizes=1
  Selector3 : Selector  InputPortWidth=6  IndexOptions=Index vector (dialog)  Indices=[2]  OutputSizes=1
  Selector4 : Selector  InputPortWidth=6  IndexOptions=Index vector (dialog)  Indices=[5]  OutputSizes=1
  Selector5 : Selector  InputPortWidth=6  IndexOptions=Index vector (dialog)  Indices=[3]  OutputSizes=1
  Selector6 : Selector  InputPortWidth=6  IndexOptions=Index vector (dialog)  Indices=[6]  OutputSizes=1
  X_6 : Outport
  wires:
  Selector6/1 -> Mux/6
  Selector5/1 -> Mux/3
  Mux/1 -> X_6/1
  Selector3/1 -> Mux/2
  Selector2/1 -> Mux/4
  Selector1/1 -> Mux/1
  Selector4/1 -> Mux/5
  X/1 -> Selector3/1, Selector5/1, Selector6/1, Selector4/1, Selector2/1, Selector1/1

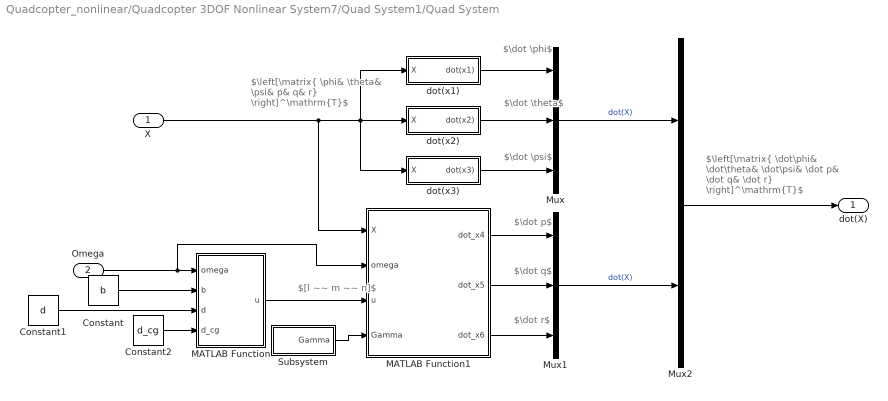
== system Quadcopter_nonlinear/Quadcopter 3DOF Nonlinear System7/Quad System1/Quad System ==
  note: $\dot \phi$
  note: $\left[\matrix{ \phi& \theta& \psi& p& q& r} \right]^\mathrm{T}$
  note: $[l ~~ m ~~ n]$
  note: $\dot \theta$
  note: $\dot \psi$
  note: $\dot p$
  note: $\dot q$
  note: $\dot r$
  note: $\left[\matrix{ \dot\phi& \dot\theta& \dot\psi& \dot p& \dot q& \dot r} \right]^\mathrm{T}$
  X : Inport
  Omega : Inport  Port=2
  Constant : Constant  Value=b
  Constant1 : Constant  Value=d
  Constant2 : Constant  Value=d_cg
  MATLAB Function : MATLAB Function  TreatAsAtomicUnit=on
  MATLAB Function1 : MATLAB Function  TreatAsAtomicUnit=on
  Mux : Mux  Inputs=3
  Mux1 : Mux  Inputs=3
  Mux2 : Mux  Inputs=2
  Subsystem : Subsystem
  dot(x1) : Subsystem
  dot(x2) : Subsystem
  dot(x3) : Subsystem
  dot(X) : Outport
  wires:
  X/1 -> MATLAB Function1/1(X), dot(x3)/1(X), dot(x1)/1(X), dot(x2)/1(X)
  Omega/1 -> MATLAB Function1/2(omega), MATLAB Function/1(omega)
  MATLAB Function1/2(dot_x5) -> Mux1/2
  dot(x2)/1(dot(x2)) -> Mux/2
  MATLAB Function1/1(dot_x4) -> Mux1/1
  dot(x3)/1(dot(x3)) -> Mux/3
  dot(x1)/1(dot(x1)) -> Mux/1
  MATLAB Function1/3(dot_x6) -> Mux1/3
  Constant/1 -> MATLAB Function/2(b)
  Constant1/1 -> MATLAB Function/3(d)
  MATLAB Function/1(u) -> MATLAB Function1/3(u)
  Mux1/1 -> Mux2/2  "dot(X)"
  Mux/1 -> Mux2/1  "dot(X)"
  Mux2/1 -> dot(X)/1
  Subsystem/1(Gamma) -> MATLAB Function1/4(Gamma)
  Constant2/1 -> MATLAB Function/4(d_cg)

== system Quadcopter_nonlinear/Quadcopter 3DOF Nonlinear System7/Quad System1/Subsystem ==
  X : Inport
  Mux : Mux  Inputs=6
  Selector1 : Selector  InputPortWidth=6  IndexOptions=Index vector (dialog)  Indices=[1]  OutputSizes=1
  Selector2 : Selector  InputPortWidth=6  IndexOptions=Index vector (dialog)  Indices=[4]  OutputSizes=1
  Selector3 : Selector  InputPortWidth=6  IndexOptions=Index vector (dialog)  Indices=[2]  OutputSizes=1
  Selector4 : Selector  InputPortWidth=6  IndexOptions=Index vector (dialog)  Indices=[5]  OutputSizes=1
  Selector5 : Selector  InputPortWidth=6  IndexOptions=Index vector (dialog)  Indices=[3]  OutputSizes=1
  Selector6 : Selector  InputPortWidth=6  IndexOptions=Index vector (dialog)  Indices=[6]  OutputSizes=1
  X_6 : Outport
  wires:
  Selector6/1 -> Mux/6
  Selector5/1 -> Mux/3
  Mux/1 -> X_6/1
  Selector3/1 -> Mux/2
  Selector2/1 -> Mux/4
  Selector1/1 -> Mux/1
  Selector4/1 -> Mux/5
  X/1 -> Selector3/1, Selector5/1, Selector6/1, Selector4/1, Selector2/1, Selector1/1

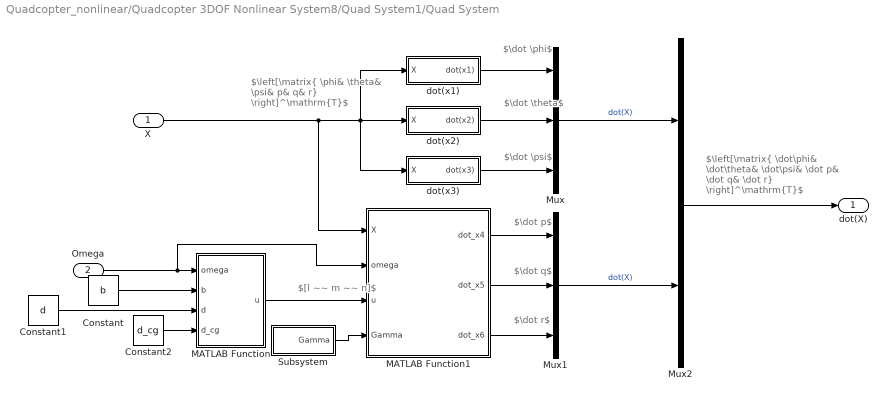
== system Quadcopter_nonlinear/Quadcopter 3DOF Nonlinear System8/Quad System1/Quad System ==
  note: $\dot \phi$
  note: $\left[\matrix{ \phi& \theta& \psi& p& q& r} \right]^\mathrm{T}$
  note: $[l ~~ m ~~ n]$
  note: $\dot \theta$
  note: $\dot \psi$
  note: $\dot p$
  note: $\dot q$
  note: $\dot r$
  note: $\left[\matrix{ \dot\phi& \dot\theta& \dot\psi& \dot p& \dot q& \dot r} \right]^\mathrm{T}$
  X : Inport
  Omega : Inport  Port=2
  Constant : Constant  Value=b
  Constant1 : Constant  Value=d
  Constant2 : Constant  Value=d_cg
  MATLAB Function : MATLAB Function  TreatAsAtomicUnit=on
  MATLAB Function1 : MATLAB Function  TreatAsAtomicUnit=on
  Mux : Mux  Inputs=3
  Mux1 : Mux  Inputs=3
  Mux2 : Mux  Inputs=2
  Subsystem : Subsystem
  dot(x1) : Subsystem
  dot(x2) : Subsystem
  dot(x3) : Subsystem
  dot(X) : Outport
  wires:
  X/1 -> MATLAB Function1/1(X), dot(x3)/1(X), dot(x1)/1(X), dot(x2)/1(X)
  Omega/1 -> MATLAB Function1/2(omega), MATLAB Function/1(omega)
  MATLAB Function1/2(dot_x5) -> Mux1/2
  dot(x2)/1(dot(x2)) -> Mux/2
  MATLAB Function1/1(dot_x4) -> Mux1/1
  dot(x3)/1(dot(x3)) -> Mux/3
  dot(x1)/1(dot(x1)) -> Mux/1
  MATLAB Function1/3(dot_x6) -> Mux1/3
  Constant/1 -> MATLAB Function/2(b)
  Constant1/1 -> MATLAB Function/3(d)
  MATLAB Function/1(u) -> MATLAB Function1/3(u)
  Mux1/1 -> Mux2/2  "dot(X)"
  Mux/1 -> Mux2/1  "dot(X)"
  Mux2/1 -> dot(X)/1
  Subsystem/1(Gamma) -> MATLAB Function1/4(Gamma)
  Constant2/1 -> MATLAB Function/4(d_cg)

== system Quadcopter_nonlinear/Quadcopter 3DOF Nonlinear System8/Quad System1/Subsystem ==
  X : Inport
  Mux : Mux  Inputs=6
  Selector1 : Selector  InputPortWidth=6  IndexOptions=Index vector (dialog)  Indices=[1]  OutputSizes=1
  Selector2 : Selector  InputPortWidth=6  IndexOptions=Index vector (dialog)  Indices=[4]  OutputSizes=1
  Selector3 : Selector  InputPortWidth=6  IndexOptions=Index vector (dialog)  Indices=[2]  OutputSizes=1
  Selector4 : Selector  InputPortWidth=6  IndexOptions=Index vector (dialog)  Indices=[5]  OutputSizes=1
  Selector5 : Selector  InputPortWidth=6  IndexOptions=Index vector (dialog)  Indices=[3]  OutputSizes=1
  Selector6 : Selector  InputPortWidth=6  IndexOptions=Index vector (dialog)  Indices=[6]  OutputSizes=1
  X_6 : Outport
  wires:
  Selector6/1 -> Mux/6
  Selector5/1 -> Mux/3
  Mux/1 -> X_6/1
  Selector3/1 -> Mux/2
  Selector2/1 -> Mux/4
  Selector1/1 -> Mux/1
  Selector4/1 -> Mux/5
  X/1 -> Selector3/1, Selector5/1, Selector6/1, Selector4/1, Selector2/1, Selector1/1

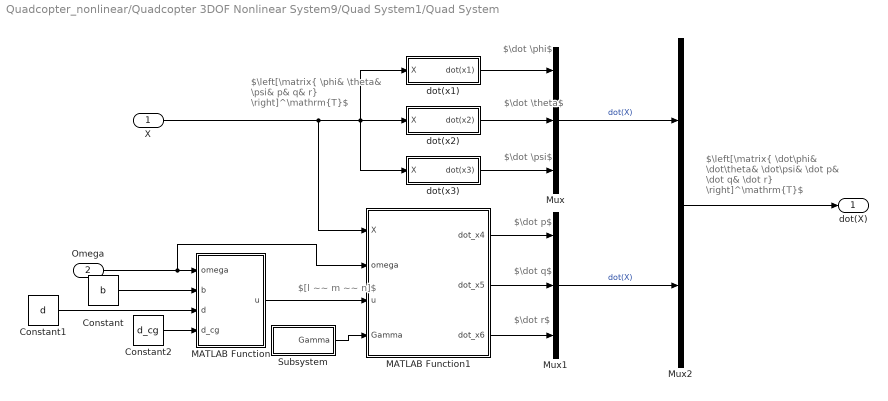
== system Quadcopter_nonlinear/Quadcopter 3DOF Nonlinear System9/Quad System1/Quad System ==
  note: $\dot \phi$
  note: $\left[\matrix{ \phi& \theta& \psi& p& q& r} \right]^\mathrm{T}$
  note: $[l ~~ m ~~ n]$
  note: $\dot \theta$
  note: $\dot \psi$
  note: $\dot p$
  note: $\dot q$
  note: $\dot r$
  note: $\left[\matrix{ \dot\phi& \dot\theta& \dot\psi& \dot p& \dot q& \dot r} \right]^\mathrm{T}$
  X : Inport
  Omega : Inport  Port=2
  Constant : Constant  Value=b
  Constant1 : Constant  Value=d
  Constant2 : Constant  Value=d_cg
  MATLAB Function : MATLAB Function  TreatAsAtomicUnit=on
  MATLAB Function1 : MATLAB Function  TreatAsAtomicUnit=on
  Mux : Mux  Inputs=3
  Mux1 : Mux  Inputs=3
  Mux2 : Mux  Inputs=2
  Subsystem : Subsystem
  dot(x1) : Subsystem
  dot(x2) : Subsystem
  dot(x3) : Subsystem
  dot(X) : Outport
  wires:
  X/1 -> MATLAB Function1/1(X), dot(x3)/1(X), dot(x1)/1(X), dot(x2)/1(X)
  Omega/1 -> MATLAB Function1/2(omega), MATLAB Function/1(omega)
  MATLAB Function1/2(dot_x5) -> Mux1/2
  dot(x2)/1(dot(x2)) -> Mux/2
  MATLAB Function1/1(dot_x4) -> Mux1/1
  dot(x3)/1(dot(x3)) -> Mux/3
  dot(x1)/1(dot(x1)) -> Mux/1
  MATLAB Function1/3(dot_x6) -> Mux1/3
  Constant/1 -> MATLAB Function/2(b)
  Constant1/1 -> MATLAB Function/3(d)
  MATLAB Function/1(u) -> MATLAB Function1/3(u)
  Mux1/1 -> Mux2/2  "dot(X)"
  Mux/1 -> Mux2/1  "dot(X)"
  Mux2/1 -> dot(X)/1
  Subsystem/1(Gamma) -> MATLAB Function1/4(Gamma)
  Constant2/1 -> MATLAB Function/4(d_cg)

== system Quadcopter_nonlinear/Quadcopter 3DOF Nonlinear System9/Quad System1/Subsystem ==
  X : Inport
  Mux : Mux  Inputs=6
  Selector1 : Selector  InputPortWidth=6  IndexOptions=Index vector (dialog)  Indices=[1]  OutputSizes=1
  Selector2 : Selector  InputPortWidth=6  IndexOptions=Index vector (dialog)  Indices=[4]  OutputSizes=1
  Selector3 : Selector  InputPortWidth=6  IndexOptions=Index vector (dialog)  Indices=[2]  OutputSizes=1
  Selector4 : Selector  InputPortWidth=6  IndexOptions=Index vector (dialog)  Indices=[5]  OutputSizes=1
  Selector5 : Selector  InputPortWidth=6  IndexOptions=Index vector (dialog)  Indices=[3]  OutputSizes=1
  Selector6 : Selector  InputPortWidth=6  IndexOptions=Index vector (dialog)  Indices=[6]  OutputSizes=1
  X_6 : Outport
  wires:
  Selector6/1 -> Mux/6
  Selector5/1 -> Mux/3
  Mux/1 -> X_6/1
  Selector3/1 -> Mux/2
  Selector2/1 -> Mux/4
  Selector1/1 -> Mux/1
  Selector4/1 -> Mux/5
  X/1 -> Selector3/1, Selector5/1, Selector6/1, Selector4/1, Selector2/1, Selector1/1

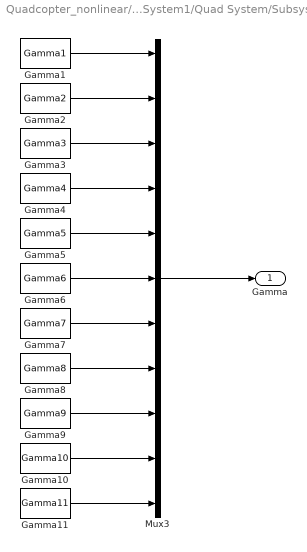
== system Quadcopter_nonlinear/Quadcopter 3DOF Nonlinear System/Quad System1/Quad System/Subsystem ==
  Gamma1 : Constant  Value=Gamma1
  Gamma10 : Constant  Value=Gamma10
  Gamma11 : Constant  Value=Gamma11
  Gamma2 : Constant  Value=Gamma2
  Gamma3 : Constant  Value=Gamma3
  Gamma4 : Constant  Value=Gamma4
  Gamma5 : Constant  Value=Gamma5
  Gamma6 : Constant  Value=Gamma6
  Gamma7 : Constant  Value=Gamma7
  Gamma8 : Constant  Value=Gamma8
  Gamma9 : Constant  Value=Gamma9
  Mux3 : Mux  Inputs=11
  Gamma : Outport
  wires:
  Gamma9/1 -> Mux3/9
  Gamma6/1 -> Mux3/6
  Mux3/1 -> Gamma/1
  Gamma8/1 -> Mux3/8
  Gamma5/1 -> Mux3/5
  Gamma7/1 -> Mux3/7
  Gamma4/1 -> Mux3/4
  Gamma3/1 -> Mux3/3
  Gamma2/1 -> Mux3/2
  Gamma1/1 -> Mux3/1
  Gamma10/1 -> Mux3/10
  Gamma11/1 -> Mux3/11

== system Quadcopter_nonlinear/Quadcopter 3DOF Nonlinear System/Quad System1/Quad System/dot(x1) ==
  X : Inport
  1 : Subsystem
  Add : Sum  Inputs=+++
  Subsystem : Subsystem
  Subsystem1 : Subsystem
  dot(x1) : Outport
  wires:
  X/1 -> Subsystem1/1(X), Subsystem/1(X), 1/1(X)  "X"
  Subsystem1/1(x4) -> Add/3
  Subsystem/1(x6cos(x1)tan(x2)) -> Add/2
  Add/1 -> dot(x1)/1
  1/1(x5sin(x1)tan(x2)) -> Add/1

== system Quadcopter_nonlinear/Quadcopter 3DOF Nonlinear System/Quad System1/Quad System/dot(x2) ==
  X : Inport
  1 : Subsystem
  Add : Sum  Inputs=+-
  Subsystem : Subsystem
  dot(x2) : Outport
  wires:
  X/1 -> Subsystem/1(X), 1/1(X)  "X"
  Subsystem/1(x6sin(x1)) -> Add/2
  Add/1 -> dot(x2)/1
  1/1(x5cos(x1)) -> Add/1

== system Quadcopter_nonlinear/Quadcopter 3DOF Nonlinear System/Quad System1/Quad System/dot(x3) ==
  X : Inport
  1 : Subsystem
  Add : Sum
  Product : Product
  Subsystem : Subsystem
  Subsystem1 : Subsystem
  dot(x3) : Outport
  wires:
  X/1 -> Subsystem1/1(X), Subsystem/1(X), 1/1(X)  "X"
  Subsystem/1(x6cos(x1)) -> Add/2
  1/1(x5sin(x1)) -> Add/1
  Product/1 -> dot(x3)/1
  Add/1 -> Product/1
  Subsystem1/1(sec(x2)) -> Product/2

== system Quadcopter_nonlinear/Quadcopter 3DOF Nonlinear System1/Quad System1/Quad System/Subsystem ==
  Gamma1 : Constant  Value=Gamma1
  Gamma10 : Constant  Value=Gamma10
  Gamma11 : Constant  Value=Gamma11
  Gamma2 : Constant  Value=Gamma2
  Gamma3 : Constant  Value=Gamma3
  Gamma4 : Constant  Value=Gamma4
  Gamma5 : Constant  Value=Gamma5
  Gamma6 : Constant  Value=Gamma6
  Gamma7 : Constant  Value=Gamma7
  Gamma8 : Constant  Value=Gamma8
  Gamma9 : Constant  Value=Gamma9
  Mux3 : Mux  Inputs=11
  Gamma : Outport
  wires:
  Gamma9/1 -> Mux3/9
  Gamma6/1 -> Mux3/6
  Mux3/1 -> Gamma/1
  Gamma8/1 -> Mux3/8
  Gamma5/1 -> Mux3/5
  Gamma7/1 -> Mux3/7
  Gamma4/1 -> Mux3/4
  Gamma3/1 -> Mux3/3
  Gamma2/1 -> Mux3/2
  Gamma1/1 -> Mux3/1
  Gamma10/1 -> Mux3/10
  Gamma11/1 -> Mux3/11

== system Quadcopter_nonlinear/Quadcopter 3DOF Nonlinear System1/Quad System1/Quad System/dot(x1) ==
  X : Inport
  1 : Subsystem
  Add : Sum  Inputs=+++
  Subsystem : Subsystem
  Subsystem1 : Subsystem
  dot(x1) : Outport
  wires:
  X/1 -> Subsystem1/1(X), Subsystem/1(X), 1/1(X)  "X"
  Subsystem1/1(x4) -> Add/3
  Subsystem/1(x6cos(x1)tan(x2)) -> Add/2
  Add/1 -> dot(x1)/1
  1/1(x5sin(x1)tan(x2)) -> Add/1

== system Quadcopter_nonlinear/Quadcopter 3DOF Nonlinear System1/Quad System1/Quad System/dot(x2) ==
  X : Inport
  1 : Subsystem
  Add : Sum  Inputs=+-
  Subsystem : Subsystem
  dot(x2) : Outport
  wires:
  X/1 -> Subsystem/1(X), 1/1(X)  "X"
  Subsystem/1(x6sin(x1)) -> Add/2
  Add/1 -> dot(x2)/1
  1/1(x5cos(x1)) -> Add/1

== system Quadcopter_nonlinear/Quadcopter 3DOF Nonlinear System1/Quad System1/Quad System/dot(x3) ==
  X : Inport
  1 : Subsystem
  Add : Sum
  Product : Product
  Subsystem : Subsystem
  Subsystem1 : Subsystem
  dot(x3) : Outport
  wires:
  X/1 -> Subsystem1/1(X), Subsystem/1(X), 1/1(X)  "X"
  Subsystem/1(x6cos(x1)) -> Add/2
  1/1(x5sin(x1)) -> Add/1
  Product/1 -> dot(x3)/1
  Add/1 -> Product/1
  Subsystem1/1(sec(x2)) -> Product/2

== system Quadcopter_nonlinear/Quadcopter 3DOF Nonlinear System2/Quad System1/Quad System/Subsystem ==
  Gamma1 : Constant  Value=Gamma1
  Gamma10 : Constant  Value=Gamma10
  Gamma11 : Constant  Value=Gamma11
  Gamma2 : Constant  Value=Gamma2
  Gamma3 : Constant  Value=Gamma3
  Gamma4 : Constant  Value=Gamma4
  Gamma5 : Constant  Value=Gamma5
  Gamma6 : Constant  Value=Gamma6
  Gamma7 : Constant  Value=Gamma7
  Gamma8 : Constant  Value=Gamma8
  Gamma9 : Constant  Value=Gamma9
  Mux3 : Mux  Inputs=11
  Gamma : Outport
  wires:
  Gamma9/1 -> Mux3/9
  Gamma6/1 -> Mux3/6
  Mux3/1 -> Gamma/1
  Gamma8/1 -> Mux3/8
  Gamma5/1 -> Mux3/5
  Gamma7/1 -> Mux3/7
  Gamma4/1 -> Mux3/4
  Gamma3/1 -> Mux3/3
  Gamma2/1 -> Mux3/2
  Gamma1/1 -> Mux3/1
  Gamma10/1 -> Mux3/10
  Gamma11/1 -> Mux3/11

== system Quadcopter_nonlinear/Quadcopter 3DOF Nonlinear System2/Quad System1/Quad System/dot(x1) ==
  X : Inport
  1 : Subsystem
  Add : Sum  Inputs=+++
  Subsystem : Subsystem
  Subsystem1 : Subsystem
  dot(x1) : Outport
  wires:
  X/1 -> Subsystem1/1(X), Subsystem/1(X), 1/1(X)  "X"
  Subsystem1/1(x4) -> Add/3
  Subsystem/1(x6cos(x1)tan(x2)) -> Add/2
  Add/1 -> dot(x1)/1
  1/1(x5sin(x1)tan(x2)) -> Add/1

== system Quadcopter_nonlinear/Quadcopter 3DOF Nonlinear System2/Quad System1/Quad System/dot(x2) ==
  X : Inport
  1 : Subsystem
  Add : Sum  Inputs=+-
  Subsystem : Subsystem
  dot(x2) : Outport
  wires:
  X/1 -> Subsystem/1(X), 1/1(X)  "X"
  Subsystem/1(x6sin(x1)) -> Add/2
  Add/1 -> dot(x2)/1
  1/1(x5cos(x1)) -> Add/1

== system Quadcopter_nonlinear/Quadcopter 3DOF Nonlinear System2/Quad System1/Quad System/dot(x3) ==
  X : Inport
  1 : Subsystem
  Add : Sum
  Product : Product
  Subsystem : Subsystem
  Subsystem1 : Subsystem
  dot(x3) : Outport
  wires:
  X/1 -> Subsystem1/1(X), Subsystem/1(X), 1/1(X)  "X"
  Subsystem/1(x6cos(x1)) -> Add/2
  1/1(x5sin(x1)) -> Add/1
  Product/1 -> dot(x3)/1
  Add/1 -> Product/1
  Subsystem1/1(sec(x2)) -> Product/2
